simulink model "actuator_models"  (R2024b)
settings: Solver=FixedStepAuto  StartTime=0.0  StopTime=4  FixedStep=0.0001  RelTol=1e-3
undefined symbols (not defined in the file or in its folder): Actuators
libraries: aerolibactuator x1
settings Model: Creator=jonno  LastModifiedBy=jonno

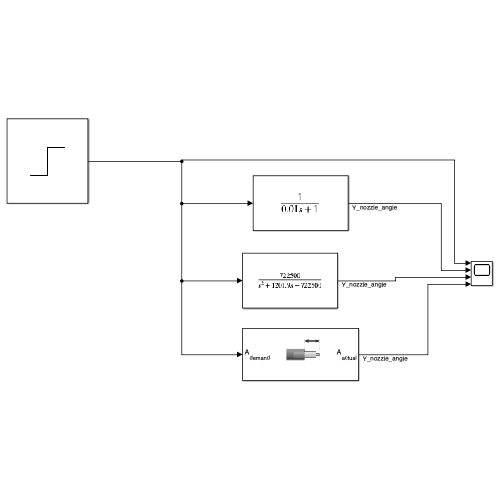
[thumbnail: Simulink's stored preview of the top-level diagram]
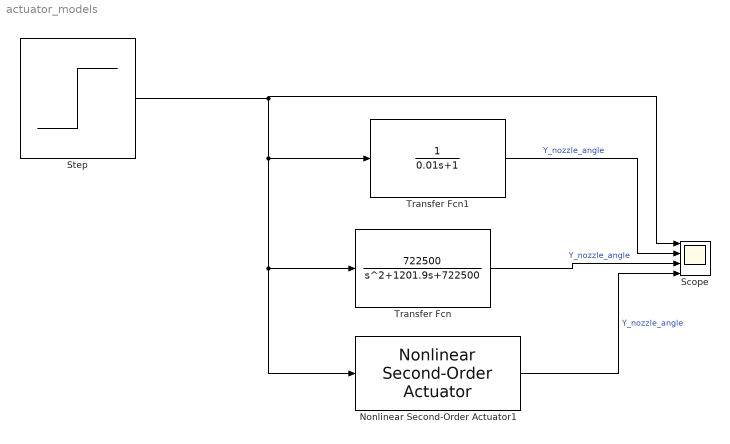
== system actuator_models ==
  Nonlinear Second-Order Actuator1 : aerolibactuator/Nonlinear Second-Order Actuator  wn_fin=Actuators.Nozzle.NaturalFreq  z_fin=Actuators.Nozzle.DampingRatio  fin_max=Actuators.Nozzle.MaxDeflection  fin_min=-Actuators.Nozzle.MaxDeflection  fin_maxrate=Actuators.Nozzle.RateLimit  fin_act_0=0  fin_act_vel=0
  Scope : Scope  NumInputPorts=4
  Step : Step  After=4*pi/180  SampleTime=0
  Transfer Fcn : TransferFcn  Numerator=[722500]  Denominator=[1 1201.9 722500]
  Transfer Fcn1 : TransferFcn  Denominator=[0.01 1]
  wires:
  Step/1 -> Nonlinear Second-Order Actuator1/1, Transfer Fcn/1, Transfer Fcn1/1, Scope/1
  Transfer Fcn/1 -> Scope/3  "Y_nozzle_angle"
  Nonlinear Second-Order Actuator1/1 -> Scope/4  "Y_nozzle_angle"
  Transfer Fcn1/1 -> Scope/2  "Y_nozzle_angle"
